simulink library "qrd_matrix_library"  (Simulink 8.7)
settings: Solver=ode45  StartTime=0.0  StopTime=10.0  RelTol=1e-3
values from neighbouring files (symbols this model uses):
  vectorization = 2    [qrd_test.m]
undefined symbols (not defined in the file or in its folder): AdvDSPBChannelOutDisplay, AdvDSPBDMemDisplay, Back_Substitution_instances, column_count, column_count_1, column_count_2, dpoly, dspba_ChannelInVis, dspba_ChannelOutVis, dspba_internal_get_channel_ports, evalAionMaskParam, latency, primtype, QRD_vectorization, recipsqrt, row, row_count, row_count_1, row_count_2, UseDontCare, value, x
libraries: DSPBAPrim x683, DSPBAControl x37, qrd_matrix_library x33, DSPBAVectorUtil x6, DSPBAVectorPrim x3
(part 5 of 8)

== system qrd_matrix_library/Back_Substitution/Sub ==
  Valid In : Inport
  Channel In : Inport  Port=2
  Acc_Data_In : Inport  Port=3
  Z_Data_In : Inport  Port=4
  ChannelIn : DSPBAPrim/ChannelIn  primtype=channelin  nInputs=dspba_internal_get_channel_ports(gcb)  nOutputs=dspba_internal_get_channel_ports(gcb)  omode=Inherit via internal rule  otype=sfix(16)  scale=2^-15  rndmethod=Unbiased  factor=1  satmethod=Symmetric  shift_vec=[0 1 2 -1]  value=2  inPortNames=['v'; 'c'; '0'; '1'; '2'; '3'; '4'; '5'; '6'; '7'; '8'; '9'; 'A'; 'B'; 'D'; 'E'; 'F'; 'G'; 'H'; 'I'; 'J'; 'K'; 'L'; 'M'; 'N'; 'O'; 'P'; 'Q'; 'R'; 'S'; 'T'; 'U'; 'W'; 'X'; 'Y'; 'Z']  outPortNames=['v'; 'c'; '0'; '1'; '2'; '3'; '4'; '5'; '6'; '7'; '8'; '9'; 'A'; 'B'; 'D'; 'E'; 'F'; 'G'; 'H'; 'I'; 'J'; 'K'; 'L'; 'M'; 'N'; 'O'; 'P'; 'Q'; 'R'; 'S'; 'T'; 'U'; 'W'; 'X'; 'Y'; 'Z']  dspbaimage=dspba_prim.jpg  text=fprintf('In');  style=Optimised  dataSignals=2  foldingEnabled=off  channels=1  sampleRate=200  packetBeginPresent=off  packetBeginEnabled=off  visibilities=dspba_ChannelInVis(gcb)  latencyCorrection=0  version=20141013
  ChannelOut : DSPBAPrim/ChannelOut  primtype=channelout  nInputs=dspba_internal_get_channel_ports(gcb)  nOutputs=dspba_internal_get_channel_ports(gcb)  omode=Inherit via internal rule  otype=sfix(16)  scale=2^-15  rndmethod=Unbiased  factor=1  satmethod=Symmetric  shift_vec=[0 1 2 -1]  value=1  inPortNames=['v'; 'c'; '0'; '1'; '2'; '3'; '4'; '5'; '6'; '7'; '8'; '9'; 'A'; 'B'; 'D'; 'E'; 'F'; 'G'; 'H'; 'I'; 'J'; 'K'; 'L'; 'M'; 'N'; 'O'; 'P'; 'Q'; 'R'; 'S'; 'T'; 'U'; 'W'; 'X'; 'Y'; 'Z']  outPortNames=['v'; 'c'; '0'; '1'; '2'; '3'; '4'; '5'; '6'; '7'; '8'; '9'; 'A'; 'B'; 'D'; 'E'; 'F'; 'G'; 'H'; 'I'; 'J'; 'K'; 'L'; 'M'; 'N'; 'O'; 'P'; 'Q'; 'R'; 'S'; 'T'; 'U'; 'W'; 'X'; 'Y'; 'Z']  dspbaimage=dspba_prim.jpg  text=fprintf('Out%s', AdvDSPBChannelOutDisplay(latency));  style=Optimised  dataSignals=1  foldingEnabled=off  channels=1  sampleRate=200  packetBeginPresent=off  packetBeginEnabled=off  visibilities=dspba_ChannelOutVis(gcb)  latency=0  latencyCorrection=0  version=20141013
  Sub : DSPBAPrim/Sub  primtype=sub  nInputs=2  nOutputs=1  omode=Inherit via internal rule with word growth  otype=sfix(16)  scale=2^-15  rndmethod=Unbiased  factor=1  satmethod=Symmetric  shift_vec=[0 1 2 -1]  value=0  inPortNames=['+'; '-';]  outPortNames=[' ']  dspbaimage=dspba_prim.jpg  text=fprintf('-');  style=Optimised  visibilities=8+2^17+2^18  floatRounding=correct  advOptions=[]  version=20130115
  SynthesisInfo : DSPBAPrim/SynthesisInfo  primtype=synthinfo  nInputs=0  nOutputs=0  omode=Inherit via internal rule  otype=sfix(16)  scale=2^-15  rndmethod=Truncate  factor=1  satmethod=Symmetric  shift_vec=[0 1 2 -1]  value=99  inPortNames=[' '; ' ';]  outPortNames=[' ']  dspbaimage=dspba_prim_ctrl.jpg  text=fprintf('Style=%s', style);  style=Scheduled  visibilities=2^17+2^18+2^19+2^20  constraintInUse=off  constraintRelation=>  constraintLimit=2  bitAccurate=off  version=20150220
  Valid_out : Outport
  Z_Acc_Data_Out : Outport  Port=2
  wires:
  ChannelIn/4 -> Sub/1
  ChannelIn/1 -> ChannelOut/1
  Z_Data_In/1 -> ChannelIn/4
  Valid In/1 -> ChannelIn/1
  Channel In/1 -> ChannelIn/2
  Acc_Data_In/1 -> ChannelIn/3
  ChannelIn/3 -> Sub/2
  Sub/1 -> ChannelOut/3
  ChannelIn/2 -> ChannelOut/2
  ChannelOut/1 -> Valid_out/1
  ChannelOut/3 -> Z_Acc_Data_Out/1

== system qrd_matrix_library/Column Major Control Logic/Address Generatioon ==
  Valid In : Inport
  Channel In : Inport  Port=2
  Iteration : Inport  Port=3
  Row Index : Inport  Port=4
  Column Index : Inport  Port=5
  Acc_Init In : Inport  Port=6
  Acc_Valid In : Inport  Port=7
  row1 : Inport  Port=8
  column1 : Inport  Port=9
  column2 : Inport  Port=10
  Done In : Inport  Port=11
  Add : DSPBAPrim/Add  primtype=add  nInputs=evalAionMaskParam(gcb,'value',1)  nOutputs=1  omode=Specify via dialog  otype=uint(nextpow2((row_count_1*column_count_1)/vectorization))  scale=1  rndmethod=Unbiased  factor=1  satmethod=Symmetric  shift_vec=[0 1 2 -1]  value=2  inPortNames=[' '; ' ';]  outPortNames=[' ']  dspbaimage=dspba_prim.jpg  text=fprintf('+');  style=Optimised  visibilities=1032+2^17+2^18+2^19  genFPC=off  floatRounding=correct  advOptions=[]  version=20130821
  Add1 : DSPBAPrim/Add  primtype=add  nInputs=evalAionMaskParam(gcb,'value',1)  nOutputs=1  omode=Specify via dialog  otype=uint(nextpow2((row_count_2*column_count_2)/vectorization))  scale=1  rndmethod=Unbiased  factor=1  satmethod=Symmetric  shift_vec=[0 1 2 -1]  value=2  inPortNames=[' '; ' ';]  outPortNames=[' ']  dspbaimage=dspba_prim.jpg  text=fprintf('+');  style=Optimised  visibilities=1032+2^17+2^18+2^19  genFPC=off  floatRounding=correct  advOptions=[]  version=20130821
  Add2 : DSPBAPrim/Add  primtype=add  nInputs=evalAionMaskParam(gcb,'value',1)  nOutputs=1  omode=Specify via dialog  otype=uint(nextpow2(row_count_1*column_count_2))  scale=1  rndmethod=Unbiased  factor=1  satmethod=Symmetric  shift_vec=[0 1 2 -1]  value=2  inPortNames=[' '; ' ';]  outPortNames=[' ']  dspbaimage=dspba_prim.jpg  text=fprintf('+');  style=Optimised  visibilities=1032+2^17+2^18+2^19  genFPC=off  floatRounding=correct  advOptions=[]  version=20130821
  ChannelIn : DSPBAPrim/ChannelIn  primtype=channelin  nInputs=dspba_internal_get_channel_ports(gcb)  nOutputs=dspba_internal_get_channel_ports(gcb)  omode=Inherit via internal rule  otype=sfix(16)  scale=2^-15  rndmethod=Unbiased  factor=1  satmethod=Symmetric  shift_vec=[0 1 2 -1]  value=9  inPortNames=['v'; 'c'; '0'; '1'; '2'; '3'; '4'; '5'; '6'; '7'; '8'; '9'; 'A'; 'B'; 'D'; 'E'; 'F'; 'G'; 'H'; 'I'; 'J'; 'K'; 'L'; 'M'; 'N'; 'O'; 'P'; 'Q'; 'R'; 'S'; 'T'; 'U'; 'W'; 'X'; 'Y'; 'Z']  outPortNames=['v'; 'c'; '0'; '1'; '2'; '3'; '4'; '5'; '6'; '7'; '8'; '9'; 'A'; 'B'; 'D'; 'E'; 'F'; 'G'; 'H'; 'I'; 'J'; 'K'; 'L'; 'M'; 'N'; 'O'; 'P'; 'Q'; 'R'; 'S'; 'T'; 'U'; 'W'; 'X'; 'Y'; 'Z']  dspbaimage=dspba_prim.jpg  text=fprintf('In');  style=Optimised  dataSignals=9  foldingEnabled=off  channels=1  sampleRate=200  packetBeginPresent=off  packetBeginEnabled=off  visibilities=dspba_ChannelInVis(gcb)  latencyCorrection=0  version=20141013
  ChannelOut : DSPBAPrim/ChannelOut  primtype=channelout  nInputs=dspba_internal_get_channel_ports(gcb)  nOutputs=dspba_internal_get_channel_ports(gcb)  omode=Inherit via internal rule  otype=sfix(16)  scale=2^-15  rndmethod=Unbiased  factor=1  satmethod=Symmetric  shift_vec=[0 1 2 -1]  value=6  inPortNames=['v'; 'c'; '0'; '1'; '2'; '3'; '4'; '5'; '6'; '7'; '8'; '9'; 'A'; 'B'; 'D'; 'E'; 'F'; 'G'; 'H'; 'I'; 'J'; 'K'; 'L'; 'M'; 'N'; 'O'; 'P'; 'Q'; 'R'; 'S'; 'T'; 'U'; 'W'; 'X'; 'Y'; 'Z']  outPortNames=['v'; 'c'; '0'; '1'; '2'; '3'; '4'; '5'; '6'; '7'; '8'; '9'; 'A'; 'B'; 'D'; 'E'; 'F'; 'G'; 'H'; 'I'; 'J'; 'K'; 'L'; 'M'; 'N'; 'O'; 'P'; 'Q'; 'R'; 'S'; 'T'; 'U'; 'W'; 'X'; 'Y'; 'Z']  dspbaimage=dspba_prim.jpg  text=fprintf('Out%s', AdvDSPBChannelOutDisplay(latency));  style=Optimised  dataSignals=6  foldingEnabled=off  channels=1  sampleRate=200  packetBeginPresent=off  packetBeginEnabled=off  visibilities=dspba_ChannelOutVis(gcb)  latency=0  latencyCorrection=0  version=20141013
  Const1 : DSPBAPrim/Const  primtype=const  nInputs=0  nOutputs=1  omode=Specify via dialog  otype=uint(8)  scale=1  rndmethod=Unbiased  factor=1  satmethod=Symmetric  shift_vec=[0 1 2 -1]  value=0  inPortNames=['+'; '+';]  outPortNames=[' ']  dspbaimage=dspba_prim.jpg  text=fprintf('%s', num2str(value));  style=Optimised  visibilities=8 + 1024  floatPrecision=float32_m23  version=20120820
  Mult : DSPBAPrim/Mult  primtype=mult  nInputs=2  nOutputs=1  omode=Inherit via internal rule  otype=sfix(16)  scale=2^-15  rndmethod=Unbiased  factor=1  satmethod=Symmetric  shift_vec=[0 1 2 -1]  value=0  inPortNames=[' '; ' ';]  outPortNames=[' ']  dspbaimage=dspba_prim.jpg  text=fprintf('X');  style=Optimised  visibilities=8+2^18+2^19  floatPrecision=float32_m23  floatRounding=correct  advOptions=[]  version=20130115
  Mult1 : DSPBAPrim/Mult  primtype=mult  nInputs=2  nOutputs=1  omode=Inherit via internal rule  otype=sfix(16)  scale=2^-15  rndmethod=Unbiased  factor=1  satmethod=Symmetric  shift_vec=[0 1 2 -1]  value=0  inPortNames=[' '; ' ';]  outPortNames=[' ']  dspbaimage=dspba_prim.jpg  text=fprintf('X');  style=Optimised  visibilities=8+2^18+2^19  floatPrecision=float32_m23  floatRounding=correct  advOptions=[]  version=20130115
  Mult2 : DSPBAPrim/Mult  primtype=mult  nInputs=2  nOutputs=1  omode=Inherit via internal rule  otype=sfix(16)  scale=2^-15  rndmethod=Unbiased  factor=1  satmethod=Symmetric  shift_vec=[0 1 2 -1]  value=0  inPortNames=[' '; ' ';]  outPortNames=[' ']  dspbaimage=dspba_prim.jpg  text=fprintf('X');  style=Optimised  visibilities=8+2^18+2^19  floatPrecision=float32_m23  floatRounding=correct  advOptions=[]  version=20130115
  SynthesisInfo : DSPBAPrim/SynthesisInfo  primtype=synthinfo  nInputs=0  nOutputs=0  omode=Inherit via internal rule  otype=sfix(16)  scale=2^-15  rndmethod=Truncate  factor=1  satmethod=Symmetric  shift_vec=[0 1 2 -1]  value=99  inPortNames=[' '; ' ';]  outPortNames=[' ']  dspbaimage=dspba_prim_ctrl.jpg  text=fprintf('Style=%s', style);  style=Scheduled  visibilities=2^17+2^18+2^19+2^20  constraintInUse=off  constraintRelation=>  constraintLimit=2  bitAccurate=off  version=20150220
  Valid Out : Outport
  Input 1 Read Address : Outport  Port=2
  Input 2 Read Address : Outport  Port=3
  Result Address : Outport  Port=4
  Acc_Init Out : Outport  Port=5
  Acc_Valid Out : Outport  Port=6
  Done Out : Outport  Port=7
  wires:
  [Done] -> ChannelOut/8
  ChannelIn/11 -> [Done]
  ChannelOut/8 -> Done Out/1
  Done In/1 -> ChannelIn/11
  ChannelIn/10 -> [Acc_Valid]
  ChannelIn/9 -> [Acc_Init]
  [Acc_Init] -> ChannelOut/6
  [Acc_Valid] -> ChannelOut/7
  Const1/1 -> ChannelOut/2
  ChannelIn/6 -> Mult2/2  "row1"
  ChannelIn/7 -> Mult/2, Mult1/2
  Acc_Valid In/1 -> ChannelIn/10
  Acc_Init In/1 -> ChannelIn/9
  ChannelIn/1 -> ChannelOut/1
  ChannelOut/7 -> Acc_Valid Out/1
  ChannelOut/6 -> Acc_Init Out/1
  column1/1 -> ChannelIn/7
  row1/1 -> ChannelIn/6
  ChannelOut/1 -> Valid Out/1
  ChannelOut/5 -> Result Address/1
  ChannelOut/4 -> Input 2 Read Address/1
  ChannelOut/3 -> Input 1 Read Address/1
  Column Index/1 -> ChannelIn/5
  Row Index/1 -> ChannelIn/4
  Iteration/1 -> ChannelIn/3
  Channel In/1 -> ChannelIn/2
  Valid In/1 -> ChannelIn/1
  Add2/1 -> ChannelOut/5  "Result Address"
  ChannelIn/4 -> Add2/2, Mult/1  "row index"
  Mult2/1 -> Add2/1
  ChannelIn/5 -> Mult2/1, Mult1/1  "column index"
  Add1/1 -> ChannelOut/4  "Input 2 Read Address"
  Add/1 -> ChannelOut/3  "Input 1 Read Address"
  ChannelIn/3 -> Add/1, Add1/1
  Mult1/1 -> Add1/2
  Mult/1 -> Add/2
  column2/1 -> ChannelIn/8

== system qrd_matrix_library/Hermitian Column Major Control Logic/Address Generatioon ==
  Valid In : Inport
  Channel In : Inport  Port=2
  Iteration : Inport  Port=3
  Column Index : Inport  Port=4
  Row Index : Inport  Port=5
  Acc_Init In : Inport  Port=6
  Acc_Valid In : Inport  Port=7
  row : Inport  Port=8
  column : Inport  Port=9
  Diagonal In : Inport  Port=10
  Done In : Inport  Port=11
  Add : DSPBAPrim/Add  primtype=add  nInputs=evalAionMaskParam(gcb,'value',1)  nOutputs=1  omode=Specify via dialog  otype=uint(nextpow2((row_count*column_count)/vectorization))  scale=1  rndmethod=Unbiased  factor=1  satmethod=Symmetric  shift_vec=[0 1 2 -1]  value=2  inPortNames=[' '; ' ';]  outPortNames=[' ']  dspbaimage=dspba_prim.jpg  text=fprintf('+');  style=Optimised  visibilities=1032+2^17+2^18+2^19  genFPC=off  floatRounding=correct  advOptions=[]  version=20130821
  Add1 : DSPBAPrim/Add  primtype=add  nInputs=evalAionMaskParam(gcb,'value',1)  nOutputs=1  omode=Specify via dialog  otype=uint(nextpow2((row_count*column_count)/vectorization))  scale=1  rndmethod=Unbiased  factor=1  satmethod=Symmetric  shift_vec=[0 1 2 -1]  value=2  inPortNames=[' '; ' ';]  outPortNames=[' ']  dspbaimage=dspba_prim.jpg  text=fprintf('+');  style=Optimised  visibilities=1032+2^17+2^18+2^19  genFPC=off  floatRounding=correct  advOptions=[]  version=20130821
  Add2 : DSPBAPrim/Add  primtype=add  nInputs=evalAionMaskParam(gcb,'value',1)  nOutputs=1  omode=Specify via dialog  otype=uint(nextpow2(row_count*row_count))  scale=1  rndmethod=Unbiased  factor=1  satmethod=Symmetric  shift_vec=[0 1 2 -1]  value=2  inPortNames=[' '; ' ';]  outPortNames=[' ']  dspbaimage=dspba_prim.jpg  text=fprintf('+');  style=Optimised  visibilities=1032+2^17+2^18+2^19  genFPC=off  floatRounding=correct  advOptions=[]  version=20130821
  Add3 : DSPBAPrim/Add  primtype=add  nInputs=evalAionMaskParam(gcb,'value',1)  nOutputs=1  omode=Specify via dialog  otype=uint(nextpow2(row_count*row_count))  scale=1  rndmethod=Unbiased  factor=1  satmethod=Symmetric  shift_vec=[0 1 2 -1]  value=2  inPortNames=[' '; ' ';]  outPortNames=[' ']  dspbaimage=dspba_prim.jpg  text=fprintf('+');  style=Optimised  visibilities=1032+2^17+2^18+2^19  genFPC=off  floatRounding=correct  advOptions=[]  version=20130821
  ChannelIn : DSPBAPrim/ChannelIn  primtype=channelin  nInputs=dspba_internal_get_channel_ports(gcb)  nOutputs=dspba_internal_get_channel_ports(gcb)  omode=Inherit via internal rule  otype=sfix(16)  scale=2^-15  rndmethod=Unbiased  factor=1  satmethod=Symmetric  shift_vec=[0 1 2 -1]  value=9  inPortNames=['v'; 'c'; '0'; '1'; '2'; '3'; '4'; '5'; '6'; '7'; '8'; '9'; 'A'; 'B'; 'D'; 'E'; 'F'; 'G'; 'H'; 'I'; 'J'; 'K'; 'L'; 'M'; 'N'; 'O'; 'P'; 'Q'; 'R'; 'S'; 'T'; 'U'; 'W'; 'X'; 'Y'; 'Z']  outPortNames=['v'; 'c'; '0'; '1'; '2'; '3'; '4'; '5'; '6'; '7'; '8'; '9'; 'A'; 'B'; 'D'; 'E'; 'F'; 'G'; 'H'; 'I'; 'J'; 'K'; 'L'; 'M'; 'N'; 'O'; 'P'; 'Q'; 'R'; 'S'; 'T'; 'U'; 'W'; 'X'; 'Y'; 'Z']  dspbaimage=dspba_prim.jpg  text=fprintf('In');  style=Optimised  dataSignals=9  foldingEnabled=off  channels=1  sampleRate=200  packetBeginPresent=off  packetBeginEnabled=off  visibilities=dspba_ChannelInVis(gcb)  latencyCorrection=0  version=20141013
  ChannelOut : DSPBAPrim/ChannelOut  primtype=channelout  nInputs=dspba_internal_get_channel_ports(gcb)  nOutputs=dspba_internal_get_channel_ports(gcb)  omode=Inherit via internal rule  otype=sfix(16)  scale=2^-15  rndmethod=Unbiased  factor=1  satmethod=Symmetric  shift_vec=[0 1 2 -1]  value=8  inPortNames=['v'; 'c'; '0'; '1'; '2'; '3'; '4'; '5'; '6'; '7'; '8'; '9'; 'A'; 'B'; 'D'; 'E'; 'F'; 'G'; 'H'; 'I'; 'J'; 'K'; 'L'; 'M'; 'N'; 'O'; 'P'; 'Q'; 'R'; 'S'; 'T'; 'U'; 'W'; 'X'; 'Y'; 'Z']  outPortNames=['v'; 'c'; '0'; '1'; '2'; '3'; '4'; '5'; '6'; '7'; '8'; '9'; 'A'; 'B'; 'D'; 'E'; 'F'; 'G'; 'H'; 'I'; 'J'; 'K'; 'L'; 'M'; 'N'; 'O'; 'P'; 'Q'; 'R'; 'S'; 'T'; 'U'; 'W'; 'X'; 'Y'; 'Z']  dspbaimage=dspba_prim.jpg  text=fprintf('Out%s', AdvDSPBChannelOutDisplay(latency));  style=Optimised  dataSignals=8  foldingEnabled=off  channels=1  sampleRate=200  packetBeginPresent=off  packetBeginEnabled=off  visibilities=dspba_ChannelOutVis(gcb)  latency=0  latencyCorrection=0  version=20141013
  Const1 : DSPBAPrim/Const  primtype=const  nInputs=0  nOutputs=1  omode=Specify via dialog  otype=uint(8)  scale=1  rndmethod=Unbiased  factor=1  satmethod=Symmetric  shift_vec=[0 1 2 -1]  value=0  inPortNames=['+'; '+';]  outPortNames=[' ']  dspbaimage=dspba_prim.jpg  text=fprintf('%s', num2str(value));  style=Optimised  visibilities=8 + 1024  floatPrecision=float32_m23  version=20120820
  Mult{,1..3} (4 alike) : DSPBAPrim/Mult  primtype=mult  nInputs=2  nOutputs=1  omode=Inherit via internal rule  otype=sfix(16)  scale=2^-15  rndmethod=Unbiased  factor=1  satmethod=Symmetric  shift_vec=[0 1 2 -1]  value=0  inPortNames=[' '; ' ';]  outPortNames=[' ']  dspbaimage=dspba_prim.jpg  text=fprintf('X');  style=Optimised  visibilities=8+2^18+2^19  floatPrecision=float32_m23  floatRounding=correct  advOptions=[]  version=20130115
  SynthesisInfo : DSPBAPrim/SynthesisInfo  primtype=synthinfo  nInputs=0  nOutputs=0  omode=Inherit via internal rule  otype=sfix(16)  scale=2^-15  rndmethod=Truncate  factor=1  satmethod=Symmetric  shift_vec=[0 1 2 -1]  value=99  inPortNames=[' '; ' ';]  outPortNames=[' ']  dspbaimage=dspba_prim_ctrl.jpg  text=fprintf('Style=%s', style);  style=Scheduled  visibilities=2^17+2^18+2^19+2^20  constraintInUse=off  constraintRelation=>  constraintLimit=2  bitAccurate=off  version=20150220
  Valid Out : Outport
  Input Transpose Read Address : Outport  Port=2
  Input Read Address : Outport  Port=3
  Result Address : Outport  Port=4
  Result Transpose Address : Outport  Port=5
  Acc_Init Out : Outport  Port=6
  Acc_Valid Out : Outport  Port=7
  Diagonal Out : Outport  Port=8
  Done Out : Outport  Port=9
  wires:
  [Done] -> ChannelOut/10
  ChannelIn/11 -> [Done]
  ChannelOut/10 -> Done Out/1
  Done In/1 -> ChannelIn/11
  ChannelIn/9 -> [Acc_Valid]
  ChannelIn/8 -> [Acc_Init]
  [Acc_Init] -> ChannelOut/7
  [Acc_Valid] -> ChannelOut/8
  [Diagonal] -> ChannelOut/9
  ChannelIn/10 -> [Diagonal]
  Const1/1 -> ChannelOut/2
  Diagonal In/1 -> ChannelIn/10
  ChannelOut/9 -> Diagonal Out/1
  ChannelIn/6 -> Mult2/2, Mult3/2
  ChannelIn/7 -> Mult/2, Mult1/2
  Acc_Valid In/1 -> ChannelIn/9
  Acc_Init In/1 -> ChannelIn/8
  ChannelIn/1 -> ChannelOut/1
  ChannelOut/8 -> Acc_Valid Out/1
  ChannelOut/7 -> Acc_Init Out/1
  column/1 -> ChannelIn/7
  row/1 -> ChannelIn/6
  ChannelOut/1 -> Valid Out/1
  ChannelOut/6 -> Result Transpose Address/1
  ChannelOut/5 -> Result Address/1
  ChannelOut/4 -> Input Read Address/1
  ChannelOut/3 -> Input Transpose Read Address/1
  Row Index/1 -> ChannelIn/5
  Column Index/1 -> ChannelIn/4
  Iteration/1 -> ChannelIn/3
  Channel In/1 -> ChannelIn/2
  Valid In/1 -> ChannelIn/1
  Add3/1 -> ChannelOut/6  "Result Transpose Address"
  Add2/1 -> ChannelOut/5  "Result Address"
  ChannelIn/4 -> Mult/1, Mult2/1, Add3/2
  Mult3/1 -> Add3/1
  Mult2/1 -> Add2/1
  ChannelIn/5 -> Mult1/1, Add2/2, Mult3/1
  Add1/1 -> ChannelOut/4  "Input Read Address"
  Add/1 -> ChannelOut/3  "Input Transpose Read Address"
  ChannelIn/3 -> Add/1, Add1/1
  Mult1/1 -> Add1/2
  Mult/1 -> Add/2

== system qrd_matrix_library/Hermitian Row Major Control Logic/Address Generatioon ==
  Valid In : Inport
  Channel In : Inport  Port=2
  Iteration : Inport  Port=3
  Row Index : Inport  Port=4
  Column Index : Inport  Port=5
  Acc_Init In : Inport  Port=6
  Acc_Valid In : Inport  Port=7
  row : Inport  Port=8
  column : Inport  Port=9
  Diagonal In : Inport  Port=10
  Done In : Inport  Port=11
  Add : DSPBAPrim/Add  primtype=add  nInputs=evalAionMaskParam(gcb,'value',1)  nOutputs=1  omode=Specify via dialog  otype=uint(nextpow2((row_count*column_count)/vectorization))  scale=1  rndmethod=Unbiased  factor=1  satmethod=Symmetric  shift_vec=[0 1 2 -1]  value=2  inPortNames=[' '; ' ';]  outPortNames=[' ']  dspbaimage=dspba_prim.jpg  text=fprintf('+');  style=Optimised  visibilities=1032+2^17+2^18+2^19  genFPC=off  floatRounding=correct  advOptions=[]  version=20130821
  Add1 : DSPBAPrim/Add  primtype=add  nInputs=evalAionMaskParam(gcb,'value',1)  nOutputs=1  omode=Specify via dialog  otype=uint(nextpow2((row_count*column_count)/vectorization))  scale=1  rndmethod=Unbiased  factor=1  satmethod=Symmetric  shift_vec=[0 1 2 -1]  value=2  inPortNames=[' '; ' ';]  outPortNames=[' ']  dspbaimage=dspba_prim.jpg  text=fprintf('+');  style=Optimised  visibilities=1032+2^17+2^18+2^19  genFPC=off  floatRounding=correct  advOptions=[]  version=20130821
  Add2 : DSPBAPrim/Add  primtype=add  nInputs=evalAionMaskParam(gcb,'value',1)  nOutputs=1  omode=Specify via dialog  otype=uint(nextpow2(row_count*row_count))  scale=1  rndmethod=Unbiased  factor=1  satmethod=Symmetric  shift_vec=[0 1 2 -1]  value=2  inPortNames=[' '; ' ';]  outPortNames=[' ']  dspbaimage=dspba_prim.jpg  text=fprintf('+');  style=Optimised  visibilities=1032+2^17+2^18+2^19  genFPC=off  floatRounding=correct  advOptions=[]  version=20130821
  Add3 : DSPBAPrim/Add  primtype=add  nInputs=evalAionMaskParam(gcb,'value',1)  nOutputs=1  omode=Specify via dialog  otype=uint(nextpow2(row_count*row_count))  scale=1  rndmethod=Unbiased  factor=1  satmethod=Symmetric  shift_vec=[0 1 2 -1]  value=2  inPortNames=[' '; ' ';]  outPortNames=[' ']  dspbaimage=dspba_prim.jpg  text=fprintf('+');  style=Optimised  visibilities=1032+2^17+2^18+2^19  genFPC=off  floatRounding=correct  advOptions=[]  version=20130821
  ChannelIn : DSPBAPrim/ChannelIn  primtype=channelin  nInputs=dspba_internal_get_channel_ports(gcb)  nOutputs=dspba_internal_get_channel_ports(gcb)  omode=Inherit via internal rule  otype=sfix(16)  scale=2^-15  rndmethod=Unbiased  factor=1  satmethod=Symmetric  shift_vec=[0 1 2 -1]  value=9  inPortNames=['v'; 'c'; '0'; '1'; '2'; '3'; '4'; '5'; '6'; '7'; '8'; '9'; 'A'; 'B'; 'D'; 'E'; 'F'; 'G'; 'H'; 'I'; 'J'; 'K'; 'L'; 'M'; 'N'; 'O'; 'P'; 'Q'; 'R'; 'S'; 'T'; 'U'; 'W'; 'X'; 'Y'; 'Z']  outPortNames=['v'; 'c'; '0'; '1'; '2'; '3'; '4'; '5'; '6'; '7'; '8'; '9'; 'A'; 'B'; 'D'; 'E'; 'F'; 'G'; 'H'; 'I'; 'J'; 'K'; 'L'; 'M'; 'N'; 'O'; 'P'; 'Q'; 'R'; 'S'; 'T'; 'U'; 'W'; 'X'; 'Y'; 'Z']  dspbaimage=dspba_prim.jpg  text=fprintf('In');  style=Optimised  dataSignals=9  foldingEnabled=off  channels=1  sampleRate=200  packetBeginPresent=off  packetBeginEnabled=off  visibilities=dspba_ChannelInVis(gcb)  latencyCorrection=0  version=20141013
  ChannelOut : DSPBAPrim/ChannelOut  primtype=channelout  nInputs=dspba_internal_get_channel_ports(gcb)  nOutputs=dspba_internal_get_channel_ports(gcb)  omode=Inherit via internal rule  otype=sfix(16)  scale=2^-15  rndmethod=Unbiased  factor=1  satmethod=Symmetric  shift_vec=[0 1 2 -1]  value=8  inPortNames=['v'; 'c'; '0'; '1'; '2'; '3'; '4'; '5'; '6'; '7'; '8'; '9'; 'A'; 'B'; 'D'; 'E'; 'F'; 'G'; 'H'; 'I'; 'J'; 'K'; 'L'; 'M'; 'N'; 'O'; 'P'; 'Q'; 'R'; 'S'; 'T'; 'U'; 'W'; 'X'; 'Y'; 'Z']  outPortNames=['v'; 'c'; '0'; '1'; '2'; '3'; '4'; '5'; '6'; '7'; '8'; '9'; 'A'; 'B'; 'D'; 'E'; 'F'; 'G'; 'H'; 'I'; 'J'; 'K'; 'L'; 'M'; 'N'; 'O'; 'P'; 'Q'; 'R'; 'S'; 'T'; 'U'; 'W'; 'X'; 'Y'; 'Z']  dspbaimage=dspba_prim.jpg  text=fprintf('Out%s', AdvDSPBChannelOutDisplay(latency));  style=Optimised  dataSignals=8  foldingEnabled=off  channels=1  sampleRate=200  packetBeginPresent=off  packetBeginEnabled=off  visibilities=dspba_ChannelOutVis(gcb)  latency=0  latencyCorrection=0  version=20141013
  Const1 : DSPBAPrim/Const  primtype=const  nInputs=0  nOutputs=1  omode=Specify via dialog  otype=uint(8)  scale=1  rndmethod=Unbiased  factor=1  satmethod=Symmetric  shift_vec=[0 1 2 -1]  value=0  inPortNames=['+'; '+';]  outPortNames=[' ']  dspbaimage=dspba_prim.jpg  text=fprintf('%s', num2str(value));  style=Optimised  visibilities=8 + 1024  floatPrecision=float32_m23  version=20120820
  Mult{,1..3} (4 alike) : DSPBAPrim/Mult  primtype=mult  nInputs=2  nOutputs=1  omode=Inherit via internal rule  otype=sfix(16)  scale=2^-15  rndmethod=Unbiased  factor=1  satmethod=Symmetric  shift_vec=[0 1 2 -1]  value=0  inPortNames=[' '; ' ';]  outPortNames=[' ']  dspbaimage=dspba_prim.jpg  text=fprintf('X');  style=Optimised  visibilities=8+2^18+2^19  floatPrecision=float32_m23  floatRounding=correct  advOptions=[]  version=20130115
  SynthesisInfo : DSPBAPrim/SynthesisInfo  primtype=synthinfo  nInputs=0  nOutputs=0  omode=Inherit via internal rule  otype=sfix(16)  scale=2^-15  rndmethod=Truncate  factor=1  satmethod=Symmetric  shift_vec=[0 1 2 -1]  value=99  inPortNames=[' '; ' ';]  outPortNames=[' ']  dspbaimage=dspba_prim_ctrl.jpg  text=fprintf('Style=%s', style);  style=Scheduled  visibilities=2^17+2^18+2^19+2^20  constraintInUse=off  constraintRelation=>  constraintLimit=2  bitAccurate=off  version=20150220
  Valid Out : Outport
  Input Transpose Read Address : Outport  Port=2
  Input Read Address : Outport  Port=3
  Result Address : Outport  Port=4
  Result Transpose Address : Outport  Port=5
  Acc_Init Out : Outport  Port=6
  Acc_Valid Out : Outport  Port=7
  Diagonal Out : Outport  Port=8
  Done Out : Outport  Port=9
  wires:
  [Done] -> ChannelOut/10
  ChannelIn/11 -> [Done]
  ChannelOut/10 -> Done Out/1
  Done In/1 -> ChannelIn/11
  ChannelIn/9 -> [Acc_Valid]
  ChannelIn/8 -> [Acc_Init]
  [Acc_Init] -> ChannelOut/7
  [Acc_Valid] -> ChannelOut/8
  [Diagonal] -> ChannelOut/9
  ChannelIn/10 -> [Diagonal]
  Const1/1 -> ChannelOut/2
  Diagonal In/1 -> ChannelIn/10
  ChannelOut/9 -> Diagonal Out/1
  ChannelIn/6 -> Mult2/2, Mult3/2
  ChannelIn/7 -> Mult/2, Mult1/2
  Acc_Valid In/1 -> ChannelIn/9
  Acc_Init In/1 -> ChannelIn/8
  ChannelIn/1 -> ChannelOut/1
  ChannelOut/8 -> Acc_Valid Out/1
  ChannelOut/7 -> Acc_Init Out/1
  column/1 -> ChannelIn/7
  row/1 -> ChannelIn/6
  ChannelOut/1 -> Valid Out/1
  ChannelOut/6 -> Result Transpose Address/1
  ChannelOut/5 -> Result Address/1
  ChannelOut/4 -> Input Read Address/1
  ChannelOut/3 -> Input Transpose Read Address/1
  Column Index/1 -> ChannelIn/5
  Row Index/1 -> ChannelIn/4
  Iteration/1 -> ChannelIn/3
  Channel In/1 -> ChannelIn/2
  Valid In/1 -> ChannelIn/1
  Add3/1 -> ChannelOut/6  "Result Transpose Address"
  Add2/1 -> ChannelOut/5  "Result Address"
  ChannelIn/4 -> Mult1/1, Mult2/1, Add3/2
  Mult3/1 -> Add3/1
  Mult2/1 -> Add2/1
  ChannelIn/5 -> Mult/1, Add2/2, Mult3/1
  Add1/1 -> ChannelOut/4  "Input Read Address"
  Add/1 -> ChannelOut/3  "Input Transpose Read Address"
  ChannelIn/3 -> Add/1, Add1/1
  Mult1/1 -> Add1/2
  Mult/1 -> Add/2

== system qrd_matrix_library/QR_decomposition/A_j ==
  Valid In : Inport
  Channel In : Inport  Port=2
  Mult_Data_In : Inport  Port=3
  A_j_Data_In : Inport  Port=4
  Aj_Address_In : Inport  Port=5
  A_j_Update_last_Valid_In : Inport  Port=6
  Done_In : Inport  Port=7
  ChannelIn : DSPBAPrim/ChannelIn  primtype=channelin  nInputs=dspba_internal_get_channel_ports(gcb)  nOutputs=dspba_internal_get_channel_ports(gcb)  omode=Inherit via internal rule  otype=sfix(16)  scale=2^-15  rndmethod=Unbiased  factor=1  satmethod=Symmetric  shift_vec=[0 1 2 -1]  value=5  inPortNames=['v'; 'c'; '0'; '1'; '2'; '3'; '4'; '5'; '6'; '7'; '8'; '9'; 'A'; 'B'; 'D'; 'E'; 'F'; 'G'; 'H'; 'I'; 'J'; 'K'; 'L'; 'M'; 'N'; 'O'; 'P'; 'Q'; 'R'; 'S'; 'T'; 'U'; 'W'; 'X'; 'Y'; 'Z']  outPortNames=['v'; 'c'; '0'; '1'; '2'; '3'; '4'; '5'; '6'; '7'; '8'; '9'; 'A'; 'B'; 'D'; 'E'; 'F'; 'G'; 'H'; 'I'; 'J'; 'K'; 'L'; 'M'; 'N'; 'O'; 'P'; 'Q'; 'R'; 'S'; 'T'; 'U'; 'W'; 'X'; 'Y'; 'Z']  dspbaimage=dspba_prim.jpg  text=fprintf('In');  style=Optimised  dataSignals=5  foldingEnabled=off  channels=1  sampleRate=200  packetBeginPresent=off  packetBeginEnabled=off  visibilities=dspba_ChannelInVis(gcb)  latencyCorrection=0  version=20141013
  ChannelOut : DSPBAPrim/ChannelOut  primtype=channelout  nInputs=dspba_internal_get_channel_ports(gcb)  nOutputs=dspba_internal_get_channel_ports(gcb)  omode=Inherit via internal rule  otype=sfix(16)  scale=2^-15  rndmethod=Unbiased  factor=1  satmethod=Symmetric  shift_vec=[0 1 2 -1]  value=4  inPortNames=['v'; 'c'; '0'; '1'; '2'; '3'; '4'; '5'; '6'; '7'; '8'; '9'; 'A'; 'B'; 'D'; 'E'; 'F'; 'G'; 'H'; 'I'; 'J'; 'K'; 'L'; 'M'; 'N'; 'O'; 'P'; 'Q'; 'R'; 'S'; 'T'; 'U'; 'W'; 'X'; 'Y'; 'Z']  outPortNames=['v'; 'c'; '0'; '1'; '2'; '3'; '4'; '5'; '6'; '7'; '8'; '9'; 'A'; 'B'; 'D'; 'E'; 'F'; 'G'; 'H'; 'I'; 'J'; 'K'; 'L'; 'M'; 'N'; 'O'; 'P'; 'Q'; 'R'; 'S'; 'T'; 'U'; 'W'; 'X'; 'Y'; 'Z']  dspbaimage=dspba_prim.jpg  text=fprintf('Out%s', AdvDSPBChannelOutDisplay(latency));  style=Optimised  dataSignals=4  foldingEnabled=off  channels=1  sampleRate=200  packetBeginPresent=off  packetBeginEnabled=off  visibilities=dspba_ChannelOutVis(gcb)  latency=0  latencyCorrection=0  version=20141013
  Sub : DSPBAPrim/Sub  primtype=sub  nInputs=2  nOutputs=1  omode=Inherit via internal rule with word growth  otype=sfix(16)  scale=2^-15  rndmethod=Unbiased  factor=1  satmethod=Symmetric  shift_vec=[0 1 2 -1]  value=0  inPortNames=['+'; '-';]  outPortNames=[' ']  dspbaimage=dspba_prim.jpg  text=fprintf('-');  style=Optimised  visibilities=8+2^17+2^18  floatRounding=correct  advOptions=[]  version=20130115
  SynthesisInfo : DSPBAPrim/SynthesisInfo  primtype=synthinfo  nInputs=0  nOutputs=0  omode=Inherit via internal rule  otype=sfix(16)  scale=2^-15  rndmethod=Truncate  factor=1  satmethod=Symmetric  shift_vec=[0 1 2 -1]  value=99  inPortNames=[' '; ' ';]  outPortNames=[' ']  dspbaimage=dspba_prim_ctrl.jpg  text=fprintf('Style=%s', style);  style=Scheduled  visibilities=2^17+2^18+2^19+2^20  constraintInUse=off  constraintRelation=>  constraintLimit=2  bitAccurate=off  version=20150220
  Valid_out : Outport
  A_j_Data_Out : Outport  Port=2
  Aj_Address_Out : Outport  Port=3
  A_j_Update_last_Valid_Out : Outport  Port=4
  Done_Out : Outport  Port=5
  wires:
  ChannelIn/4 -> Sub/1
  ChannelIn/1 -> ChannelOut/1
  A_j_Data_In/1 -> ChannelIn/4
  Valid In/1 -> ChannelIn/1
  Channel In/1 -> ChannelIn/2
  Mult_Data_In/1 -> ChannelIn/3
  ChannelIn/3 -> Sub/2
  Sub/1 -> ChannelOut/3
  ChannelIn/2 -> ChannelOut/2
  ChannelOut/1 -> Valid_out/1
  ChannelOut/3 -> A_j_Data_Out/1
  Aj_Address_In/1 -> ChannelIn/5
  ChannelOut/4 -> Aj_Address_Out/1
  ChannelIn/5 -> ChannelOut/4
  A_j_Update_last_Valid_In/1 -> ChannelIn/6
  ChannelOut/5 -> A_j_Update_last_Valid_Out/1
  ChannelIn/6 -> ChannelOut/5
  Done_In/1 -> ChannelIn/7
  ChannelOut/6 -> Done_Out/1
  ChannelIn/7 -> ChannelOut/6

== system qrd_matrix_library/QR_decomposition/A_k Memory Controller ==
  Write_Enable : Inport
  Write_Address : Inport  Port=2
  Write_Data : Inport  Port=3
  A_k_Read_Valid1 : Inport  Port=4
  A_k_Read_Address1 : Inport  Port=5
  A_k_Read_Valid2 : Inport  Port=6
  A_k_Read_Address2 : Inport  Port=7
  A_k_Read_Valid3 : Inport  Port=8
  A_k_Read_Address3 : Inport  Port=9
  A_k Memory : DSPBAPrim/DualMem  primtype=dualmem  nInputs=4  nOutputs=2  omode=single  otype=sfix(16)  scale=2^-15  rndmethod=Unbiased  factor=1  satmethod=Symmetric  shift_vec=[0 1 2 -1]  value=complex(zeros(size/vectorization,vectorization),zeros(size/vectorization,vectorization))  inPortNames=['d1'; 'a1'; 'w1'; 'a2']  outPortNames=['q1'; 'q2']  dspbaimage=dspba_prim.jpg  text=fprintf('dmem%s',AdvDSPBDMemDisplay(UseDontCare));  style=Optimised  visibilities=8 + 1024 + 2^17 + 2^18  UseDontCare=off  TwinWritePorts=off  version=20141001
  A_k Memory Read Address Select : DSPBAPrim/Select  primtype=select  nInputs=str2num(get_param(gcb,'value'))*2+1  nOutputs=1  omode=Inherit via internal rule  otype=sfix(16)  scale=2^-15  rndmethod=Unbiased  factor=1  satmethod=Symmetric  shift_vec=[0 1 2 -1]  value=3  inPortNames=['d'; '0'; 'a'; '1'; 'b'; '2'; 'c'; '3'; 'd'; '4'; 'e'; '5'; 'f'; '6'; 'g'; '7'; 'h'; '8'; 'i'; '9'; 'j']  outPortNames=[' ']  dspbaimage=dspba_prim.jpg  text=fprintf('%s', primtype);  style=Optimised  visibilities=8 + 1024  version=20090407
  Read_Data : Outport
  wires:
  Write_Address/1 -> A_k Memory/2
  Write_Enable/1 -> A_k Memory/3
  Write_Data/1 -> A_k Memory/1
  A_k Memory/2 -> Read_Data/1
  A_k_Read_Address1/1 -> A_k Memory Read Address Select/1, A_k Memory Read Address Select/3
  A_k_Read_Valid2/1 -> A_k Memory Read Address Select/4
  A_k_Read_Address2/1 -> A_k Memory Read Address Select/5
  A_k_Read_Valid1/1 -> A_k Memory Read Address Select/2
  A_k Memory Read Address Select/1 -> A_k Memory/4
  A_k_Read_Address3/1 -> A_k Memory Read Address Select/7
  A_k_Read_Valid3/1 -> A_k Memory Read Address Select/6

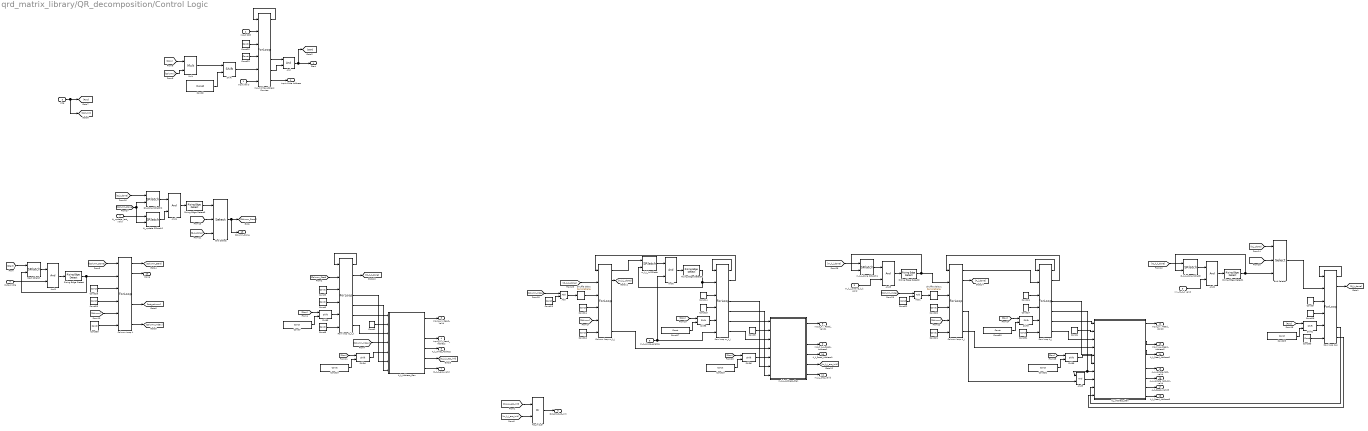
== system qrd_matrix_library/QR_decomposition/Control Logic ==
  Input Valid : Inport
  Input SOP : Inport  Port=2
  size : Inport  Port=3
  Output Idle : Inport  Port=4
  inv_r2_k_k valid : Inport  Port=5
  rn_k_j_over_r2_k_k valid : Inport  Port=6
  Aj_update_last_valid : Inport  Port=7
  rn_k_j_loop_enable : Inport  Port=8
  A_j_Address_Gen : Subsystem
  A_k_Address_Gen : Subsystem
  Acc_Init_Or : DSPBAPrim/Or  primtype=or  nInputs=2  nOutputs=1  omode=Inherit via internal rule  otype=sfix(16)  scale=2^-15  rndmethod=Unbiased  factor=1  satmethod=Symmetric  shift_vec=[0 1 2 -1]  value=0  inPortNames=[' '; ' '; ' '; ' '; ' '; ' '; ' '; ' '; ' '; ' '; ' '; ' '; ' '; ' '; ' '; ' '; ]  outPortNames=[' ']  dspbaimage=dspba_prim.jpg  text=fprintf('|');  style=Optimised  visibilities=8+2  version=20090407
  Add : DSPBAPrim/Add  primtype=add  nInputs=evalAionMaskParam(gcb,'value',1)  nOutputs=1  omode=Inherit via internal rule with word growth  otype=uint(nextpow2(row_count*row_count))  scale=1  rndmethod=Unbiased  factor=1  satmethod=Symmetric  shift_vec=[0 1 2 -1]  value=2  inPortNames=[' '; ' ';]  outPortNames=[' ']  dspbaimage=dspba_prim.jpg  text=fprintf('+');  style=Optimised  visibilities=1032+2^17+2^18+2^19  genFPC=off  floatRounding=correct  advOptions=[]  version=20130821
  Add1 : DSPBAPrim/Add  primtype=add  nInputs=evalAionMaskParam(gcb,'value',1)  nOutputs=1  omode=Inherit via internal rule with word growth  otype=uint(nextpow2(row_count*row_count))  scale=1  rndmethod=Unbiased  factor=1  satmethod=Symmetric  shift_vec=[0 1 2 -1]  value=2  inPortNames=[' '; ' ';]  outPortNames=[' ']  dspbaimage=dspba_prim.jpg  text=fprintf('+');  style=Optimised  visibilities=1032+2^17+2^18+2^19  genFPC=off  floatRounding=correct  advOptions=[]  version=20130821
  Aj_update SRlatch2 : DSPBAControl/SRlatch
  And{,1..6} (7 alike) : DSPBAPrim/And  primtype=and  nInputs=2  nOutputs=1  omode=Inherit via internal rule  otype=sfix(16)  scale=2^-15  rndmethod=Unbiased  factor=1  satmethod=Symmetric  shift_vec=[0 1 2 -1]  value=0  inPortNames=[' '; ' '; ' '; ' '; ' '; ' '; ' '; ' '; ' '; ' '; ' '; ' '; ' '; ' '; ' '; ' '; ]  outPortNames=[' ']  dspbaimage=dspba_prim.jpg  text=fprintf('&');  style=Optimised  visibilities=8+2  version=20090407
  Column Loop k : DSPBAPrim/ForLoop  looptest=<
  Column loop A_j : DSPBAPrim/ForLoop  looptest=<
  Column loop rn_k_j : DSPBAPrim/ForLoop  looptest=<
  Const1 : DSPBAPrim/Const  primtype=const  nInputs=0  nOutputs=1  omode=Specify via dialog  otype=uint(8)  scale=1  rndmethod=Unbiased  factor=1  satmethod=Symmetric  shift_vec=[0 1 2 -1]  value=0  inPortNames=['+'; '+';]  outPortNames=[' ']  dspbaimage=dspba_prim.jpg  text=fprintf('%s', num2str(value));  style=Optimised  visibilities=8 + 1024  floatPrecision=float32_m23  version=20120820
  Const{2,7,10,17,19,29..30,32} (8 alike) : DSPBAPrim/Const  primtype=const  nInputs=0  nOutputs=1  omode=Inherit via internal rule  otype=uint(8)  scale=1  rndmethod=Unbiased  factor=1  satmethod=Symmetric  shift_vec=[0 1 2 -1]  value=nextpow2(vectorization)  inPortNames=['+'; '+';]  outPortNames=[' ']  dspbaimage=dspba_prim.jpg  text=fprintf('%s', num2str(value));  style=Optimised  visibilities=8 + 1024  floatPrecision=float32_m23  version=20120820
  Const{6,8,11..13,15..16,20..23,26..27,31,33,35} (16 alike) : DSPBAPrim/Const  primtype=const  nInputs=0  nOutputs=1  omode=Inherit via internal rule  otype=uint(8)  scale=1  rndmethod=Unbiased  factor=1  satmethod=Symmetric  shift_vec=[0 1 2 -1]  value=1  inPortNames=['+'; '+';]  outPortNames=[' ']  dspbaimage=dspba_prim.jpg  text=fprintf('%s', num2str(value));  style=Optimised  visibilities=8 + 1024  floatPrecision=float32_m23  version=20120820
  Const{5,9,14,24..25,28} (6 alike) : DSPBAPrim/Const  primtype=const  nInputs=0  nOutputs=1  omode=Inherit via internal rule  otype=uint(8)  scale=1  rndmethod=Unbiased  factor=1  satmethod=Symmetric  shift_vec=[0 1 2 -1]  value=0  inPortNames=['+'; '+';]  outPortNames=[' ']  dspbaimage=dspba_prim.jpg  text=fprintf('%s', num2str(value));  style=Optimised  visibilities=8 + 1024  floatPrecision=float32_m23  version=20120820
  Const3 : DSPBAPrim/Const  primtype=const  nInputs=0  nOutputs=1  omode=Specify via dialog  otype=uint(8)  scale=1  rndmethod=Unbiased  factor=1  satmethod=Symmetric  shift_vec=[0 1 2 -1]  value=0  inPortNames=['+'; '+';]  outPortNames=[' ']  dspbaimage=dspba_prim.jpg  text=fprintf('%s', num2str(value));  style=Optimised  visibilities=8 + 1024  floatPrecision=float32_m23  version=20120820
  Const4 : DSPBAPrim/Const  primtype=const  nInputs=0  nOutputs=1  omode=Specify via dialog  otype=uint(8)  scale=1  rndmethod=Unbiased  factor=1  satmethod=Symmetric  shift_vec=[0 1 2 -1]  value=0  inPortNames=['+'; '+';]  outPortNames=[' ']  dspbaimage=dspba_prim.jpg  text=fprintf('%s', num2str(value));  style=Optimised  visibilities=8 + 1024  floatPrecision=float32_m23  version=20120820
  End Select : DSPBAPrim/Select  primtype=select  nInputs=str2num(get_param(gcb,'value'))*2+1  nOutputs=1  omode=Inherit via internal rule  otype=sfix(16)  scale=2^-15  rndmethod=Unbiased  factor=1  satmethod=Symmetric  shift_vec=[0 1 2 -1]  value=1  inPortNames=['d'; '0'; 'a'; '1'; 'b'; '2'; 'c'; '3'; 'd'; '4'; 'e'; '5'; 'f'; '6'; 'g'; '7'; 'h'; '8'; 'i'; '9'; 'j']  outPortNames=[' ']  dspbaimage=dspba_prim.jpg  text=fprintf('%s', primtype);  style=Optimised  visibilities=8 + 1024  version=20090407
  End Select1 : DSPBAPrim/Select  primtype=select  nInputs=str2num(get_param(gcb,'value'))*2+1  nOutputs=1  omode=Inherit via internal rule  otype=sfix(16)  scale=2^-15  rndmethod=Unbiased  factor=1  satmethod=Symmetric  shift_vec=[0 1 2 -1]  value=1  inPortNames=['d'; '0'; 'a'; '1'; 'b'; '2'; 'c'; '3'; 'd'; '4'; 'e'; '5'; 'f'; '6'; 'g'; '7'; 'h'; '8'; 'i'; '9'; 'j']  outPortNames=[' ']  dspbaimage=dspba_prim.jpg  text=fprintf('%s', primtype);  style=Optimised  visibilities=8 + 1024  version=20090407
  Input Write Address Counter : DSPBAPrim/ForLoop  looptest=<
  Mult : DSPBAPrim/Mult  primtype=mult  nInputs=2  nOutputs=1  omode=Inherit via internal rule  otype=sfix(16)  scale=2^-15  rndmethod=Unbiased  factor=1  satmethod=Symmetric  shift_vec=[0 1 2 -1]  value=0  inPortNames=[' '; ' ';]  outPortNames=[' ']  dspbaimage=dspba_prim.jpg  text=fprintf('X');  style=Optimised  visibilities=8+2^18+2^19  floatPrecision=float32_m23  floatRounding=correct  advOptions=[]  version=20130115
  Qk_done SRlatch2 : DSPBAControl/SRlatch
  Rising Edge Detect{,1..4} (5 alike) : qrd_matrix_library/hermitian_matrix_multiplication/Rising Edge Detect
  Row loop A_j : DSPBAPrim/ForLoop  looptest=<
  Row loop Q_k : DSPBAPrim/ForLoop  looptest=<
  Row loop r2_k_k : DSPBAPrim/ForLoop  looptest=<
  Row loop rn_k_j : DSPBAPrim/ForLoop  looptest=<
  Shift{,1,3..8} (8 alike) : DSPBAPrim/Shift  primtype=shift  nInputs=2  nOutputs=1  omode=Inherit via internal rule  otype=sfix(16)  scale=2^-15  rndmethod=Unbiased  factor=1  satmethod=Symmetric  shift_vec=[0 1 2 -1]  value=0  inPortNames=['a'; 'b';]  outPortNames=[' ']  dspbaimage=dspba_prim.jpg  text=fprintf('a >> b');  style=Optimised  visibilities=8  version=20090407
  Shuffle delay : DSPBAPrim/SampleDelay  primtype=sampdelay  nInputs=1  nOutputs=1  omode=Inherit via internal rule  otype=sfix(16)  scale=2^-15  rndmethod=Unbiased  factor=1  satmethod=Symmetric  shift_vec=[0 1 2 -1]  value=1  inPortNames=[' '; ' ';]  outPortNames=[' ']  dspbaimage=dspba_prim.jpg  text=dpoly(1, eye(1,value+1), 'z')  style=Optimised  visibilities=8 + 1024 + 2^17 + 2^18  flexible=off  slackgroup=0  augmented=0  version=20090407  advOptions=[]
  Shuffle delay1 : DSPBAPrim/SampleDelay  primtype=sampdelay  nInputs=1  nOutputs=1  omode=Inherit via internal rule  otype=sfix(16)  scale=2^-15  rndmethod=Unbiased  factor=1  satmethod=Symmetric  shift_vec=[0 1 2 -1]  value=1  inPortNames=[' '; ' ';]  outPortNames=[' ']  dspbaimage=dspba_prim.jpg  text=dpoly(1, eye(1,value+1), 'z')  style=Optimised  visibilities=8 + 1024 + 2^17 + 2^18  flexible=off  slackgroup=0  augmented=0  version=20090407  advOptions=[]
  Start SRlatch : DSPBAControl/SRlatch
  r2_k_k_done SRlatch : DSPBAControl/SRlatch
  rn_k_j_Address_Gen : Subsystem
  rn_k_j_done SRlatch1 : DSPBAControl/SRlatch
  rn_k_j_ls SRlatch : DSPBAControl/SRlatch
  Start : Outport
  Input Write Address : Outport  Port=2
  Input_A_k_Read_Valid : Outport  Port=3
  Input_A_k_Read_Address : Outport  Port=4
  A_k_Write_Address : Outport  Port=5
  Dot_Product_Init : Outport  Port=6
  r2_k_k_acc_valid : Outport  Port=7
  Input_A_j_Read_Valid1 : Outport  Port=8
  Input_A_j_Read_Address1 : Outport  Port=9
  A_k_Read_Address1 : Outport  Port=10
  rn_k_j_acc_valid : Outport  Port=11
  Input_A_j_Read_Valid2 : Outport  Port=12
  Input_A_j_Read_Address2 : Outport  Port=13
  A_k_Read_Address2 : Outport  Port=14
  A_j_update_last_valid : Outport  Port=15
  A_j_update_last_col_valid : Outport  Port=16
  A_k_Read_Valid3 : Outport  Port=17
  A_k_Read_Address3 : Outport  Port=18
  Column_Done : Outport  Port=19
  Done : Outport  Port=20
  wires:
  Rising Edge Detect/1 -> Column Loop k/2, Start SRlatch/2
  And1/1 -> Rising Edge Detect/1
  Output Idle/1 -> And1/2
  Start SRlatch/1 -> And1/1
  Shift/1 -> Input Write Address Counter/5
  Const23/1 -> Input Write Address Counter/4
  Const25/1 -> Input Write Address Counter/3
  Input Write Address Counter/7 -> Input Write Address/1
  [Column] -> Column Loop k/5
  Const26/1 -> Column Loop k/4
  Const28/1 -> Column Loop k/3
  [Start] -> Start SRlatch/1
  Column Loop k/7 -> [Column_Index]
  Const35/1 -> Column Loop k/6
  [Column_Done] -> Column Loop k/1
  Column Loop k/1 -> [Column_Start]
  Column Loop k/2 -> Done/1
  size/1 -> [Column], [Row]
  [Row] -> Mult/1
  [Column] -> Mult/2
  Mult/1 -> Shift/1
  Const2/1 -> Shift/2
  Input Valid/1 -> Input Write Address Counter/6
  Input Write Address Counter/1 -> Input Write Address Counter/1
  And/1 -> [Start], Start/1
  Input Write Address Counter/5 -> And/1
  Input Write Address Counter/6 -> And/2
  Input SOP/1 -> Input Write Address Counter/2
  [Column_Start] -> Row loop r2_k_k/2
  Const5/1 -> Row loop r2_k_k/3
  Const6/1 -> Row loop r2_k_k/4
  Shift3/1 -> Row loop r2_k_k/5
  [Row] -> Shift3/1
  Const7/1 -> Shift3/2
  Const8/1 -> Row loop r2_k_k/6
  Row loop r2_k_k/1 -> Row loop r2_k_k/1
  Row loop r2_k_k/6 -> A_k_Address_Gen/1(Valid_In)
  Row loop r2_k_k/7 -> A_k_Address_Gen/3(Row_Index)
  A_k_Address_Gen/3(Input_Read_Address) -> Input_A_k_Read_Address/1
  A_k_Address_Gen/1(Valid_Out) -> Input_A_k_Read_Valid/1
  Const1/1 -> A_k_Address_Gen/2(Channel_In)
  [Column_Index] -> A_k_Address_Gen/4(Column)
  [Row] -> Shift4/1
  Const10/1 -> Shift4/2
  Shift4/1 -> A_k_Address_Gen/5(Row)
  Row loop r2_k_k/4 -> A_k_Address_Gen/6(Acc_Init_In)
  Row loop r2_k_k/5 -> A_k_Address_Gen/7(Acc_Valid_In)
  A_k_Address_Gen/5(Acc_Init_Out) -> [r2_k_k_acc_init]
  Row loop r2_k_k/2 -> [r2_k_k_done]
  A_k_Address_Gen/4(A_k_Write_Address) -> A_k_Write_Address/1
  [r2_k_k_acc_init] -> Acc_Init_Or/1
  [rn_k_j_acc_init] -> Acc_Init_Or/2
  Acc_Init_Or/1 -> Dot_Product_Init/1
  A_k_Address_Gen/6(Acc_Valid_Out) -> r2_k_k_acc_valid/1
  Const11/1 -> Column loop rn_k_j/4
  [Column] -> Column loop rn_k_j/5
  Const12/1 -> Column loop rn_k_j/6
  [Column_Index] -> Add/1
  Add/1 -> Shuffle delay/1
  Const13/1 -> Add/2
  Column loop rn_k_j/1 -> rn_k_j_ls SRlatch/1
  Const14/1 -> Row loop rn_k_j/3
  Const15/1 -> Row loop rn_k_j/4
  Shift5/1 -> Row loop rn_k_j/5
  [Row] -> Shift5/1
  Const17/1 -> Shift5/2
  rn_k_j_loop_enable/1 -> And6/2, Row loop rn_k_j/6
  Row loop rn_k_j/1 -> Row loop rn_k_j/1
  Row loop rn_k_j/2 -> Column loop rn_k_j/1
  Column loop rn_k_j/2 -> [rn_k_j_done]
  Row loop rn_k_j/6 -> rn_k_j_Address_Gen/1(Valid_In)
  Const3/1 -> rn_k_j_Address_Gen/2(Channel_In)
  Row loop rn_k_j/7 -> rn_k_j_Address_Gen/3(Row_Index)
  Column loop rn_k_j/7 -> rn_k_j_Address_Gen/4(Column)
  [Row] -> Shift6/1
  Const19/1 -> Shift6/2
  Shift6/1 -> rn_k_j_Address_Gen/5(Row)
  Row loop rn_k_j/4 -> rn_k_j_Address_Gen/6(Acc_Init_In)
  Row loop rn_k_j/5 -> rn_k_j_Address_Gen/7(Acc_Valid_In)
  rn_k_j_Address_Gen/1(Valid_Out) -> Input_A_j_Read_Valid1/1
  rn_k_j_Address_Gen/3(A_k_j_Read_Address) -> Input_A_j_Read_Address1/1
  rn_k_j_Address_Gen/4(A_k_Read_Address) -> A_k_Read_Address1/1
  rn_k_j_Address_Gen/5(Acc_Init_Out) -> [rn_k_j_acc_init]
  rn_k_j_Address_Gen/6(Acc_Valid_Out) -> rn_k_j_acc_valid/1
  Shuffle delay/1 -> Column loop rn_k_j/3
  [r2_k_k_done] -> r2_k_k_done SRlatch/1
  And2/1 -> Rising Edge Detect1/1
  r2_k_k_done SRlatch/1 -> And2/1
  Rising Edge Detect2/1 -> Column loop A_j/2, rn_k_j_done SRlatch1/2
  Const20/1 -> Column loop A_j/4
  [Column] -> Column loop A_j/5
  Const21/1 -> Column loop A_j/6
  [Column_Index] -> Add1/1
  Add1/1 -> Shuffle delay1/1
  Const22/1 -> Add1/2
  Column loop A_j/1 -> Row loop A_j/2
  Const24/1 -> Row loop A_j/3
  Const27/1 -> Row loop A_j/4
  Shift7/1 -> Row loop A_j/5
  [Row] -> Shift7/1
  Const30/1 -> Shift7/2
  Const31/1 -> Row loop A_j/6
  Row loop A_j/1 -> Row loop A_j/1
  Row loop A_j/2 -> Column loop A_j/1
  Column loop A_j/2 -> [A_j_done]
  Row loop A_j/6 -> A_j_Address_Gen/1(Valid_In)
  Const4/1 -> A_j_Address_Gen/2(Channel_In)
  Row loop A_j/7 -> A_j_Address_Gen/3(Row_Index)
  Column loop A_j/7 -> A_j_Address_Gen/4(Column)
  [Row] -> Shift8/1
  Const32/1 -> Shift8/2
  Shift8/1 -> A_j_Address_Gen/5(Row)
  Row loop A_j/4 -> A_j_Address_Gen/6(Acc_Init_In)
  Row loop A_j/5 -> And5/1, A_j_Address_Gen/7(Acc_Valid_In)
  A_j_Address_Gen/1(Valid_Out) -> Input_A_j_Read_Valid2/1
  A_j_Address_Gen/3(A_k_j_Read_Address) -> Input_A_j_Read_Address2/1
  A_j_Address_Gen/4(A_k_Read_Address) -> A_k_Read_Address2/1
  A_j_Address_Gen/6(Acc_Valid_Out) -> A_j_update_last_valid/1
  [rn_k_j_done] -> rn_k_j_done SRlatch1/1
  And3/1 -> Rising Edge Detect2/1
  rn_k_j_done SRlatch1/1 -> And3/1
  rn_k_j_over_r2_k_k valid/1 -> And3/2
  Shuffle delay1/1 -> Column loop A_j/3
  [Q_k_done] -> Qk_done SRlatch2/1
  And4/1 -> Rising Edge Detect3/1
  Qk_done SRlatch2/1 -> And4/1
  Aj_update_last_valid/1 -> Aj_update SRlatch2/1
  inv_r2_k_k valid/1 -> And2/2
  Row loop Q_k/1 -> Row loop Q_k/1
  [Row] -> Shift1/1
  Const29/1 -> Shift1/2
  Const33/1 -> Row loop Q_k/6
  Shift1/1 -> Row loop Q_k/5
  Const16/1 -> Row loop Q_k/4
  Const9/1 -> Row loop Q_k/3
  Row loop Q_k/2 -> [Q_k_done]
  Aj_update SRlatch2/1 -> And4/2
  A_j_Address_Gen/9(A_k_Read_Address3_Out) -> A_k_Read_Address3/1
  A_j_Address_Gen/8(A_k_Read_Valid3_Out) -> A_k_Read_Valid3/1
  Row loop Q_k/6 -> A_j_Address_Gen/9(A_k_Read_Valid3_In)
  Row loop Q_k/7 -> A_j_Address_Gen/10(A_k_Read_Address3_In)
  End Select/1 -> Column_Done/1, [Column_Done]
  Rising Edge Detect3/1 -> End Select/1
  Column Loop k/5 -> [last_column]
  [last_column] -> End Select/2
  [Q_k_done] -> End Select/3
  [Column_Done] -> Aj_update SRlatch2/2, Qk_done SRlatch2/2
  A_j_Address_Gen/7(Aj_last_col_update_out) -> A_j_update_last_col_valid/1
  And5/1 -> A_j_Address_Gen/8(Aj_last_col_update_in)
  Column loop A_j/5 -> And5/2
  [last_column] -> End Select1/2
  Rising Edge Detect1/1 -> End Select1/3, r2_k_k_done SRlatch/2
  [A_j_done] -> End Select1/1
  End Select1/1 -> Row loop Q_k/2
  [r2_k_k_done] -> Column loop rn_k_j/2
  And6/1 -> Rising Edge Detect4/1
  rn_k_j_ls SRlatch/1 -> And6/1
  Rising Edge Detect4/1 -> Row loop rn_k_j/2, rn_k_j_ls SRlatch/2
